simulink model "Comp_FDC_main"  (R2021b)
settings: Solver=FixedStepDiscrete  StartTime=0.0  StopTime=10.0  RelTol=1e-3  EnableMultiTasking=on
settings Model: DataDictionary=APPTypes.sldd  Creator=FVT23010  LastModifiedBy=FVT23010
settings SolverCC: AutoInsertRateTranBlk=on
settings DataIOCC: SaveFormat=StructureWithTime
settings OptimizationCC: DefaultParameterBehavior=Inlined  EnhancedBackFolding=on  PassReuseOutputArgsAs=Individual arguments  ZeroExternalMemoryAtStartup=off  ZeroInternalMemoryAtStartup=off  OptimizeBlockOrder=speed  DifferentSizesBufferReuse=on  OptimizationCustomize=off  EfficientTunableParamExpr=on
settings DebuggingCC: ParameterTunabilityLossMsg=error
settings ModelReferenceCC: ModelReferenceNumInstancesAllowed=Single
settings SFSimCC: MATLABDynamicMemAlloc=off
settings RTWCC: Description=AUTOSAR  SystemTargetFile=autosar.tlc  GenCodeOnly=on  TemplateMakefile=ert_default_tmf
settings CodeAppCC: ForceParamTrailComments=on  IgnoreCustomStorageClasses=off  OperatorAnnotations=on  SimulinkDataObjDesc=on  SFDataObjDesc=on  InsertBlockDesc=on
settings STFCustomTargetCC: TargetLangStandard=C99 (ISO)  MultiwordLength=256  ParMdlRefBuildCompliant=on  CompOptLevelCompliant=on  IncludeMdlTerminateFcn=off  CombineOutputUpdateFcns=on  SuppressErrorStatus=on  ERTCustomFileBanners=on  SupportNonFinite=off  SupportComplex=off  SupportContinuousTime=off  SupportNonInlinedSFcns=off  RemoveResetFunc=on  MATLABClassNameForMDSCustomization=Simulink.SoftwareTarget.ERTCustomization  AutosarCompliant=on  GRTInterface=off  UseToolchainInfoCompliant=on  LookupTableObjectStructAxisOrder=2,1,3,4,...  LUTObjectStructOrderEvenSpacing=Size,Table,Breakpoints  SystemTargetFile=autosar.tlc
settings ERTTargetCC: TargetLangStandard=C99 (ISO)  ConcurrentExecutionCompliant=off  IncludeMdlTerminateFcn=off  SuppressErrorStatus=on  SupportNonFinite=off  SupportComplex=off  ModelStepFunctionPrototypeControlCompliant=off  CPPClassGenCompliant=off  AutosarCompliant=on  LookupTableObjectStructAxisOrder=2,1,3,4,...  LUTObjectStructOrderEvenSpacing=Size,Table,Breakpoints  InlinedParameterPlacement=NonHierarchical  ERTCustomFileTemplate=example_file_process.tlc

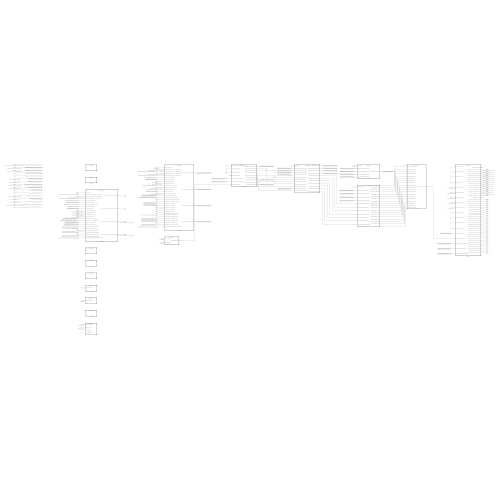
[thumbnail: Simulink's stored preview of the top-level diagram]
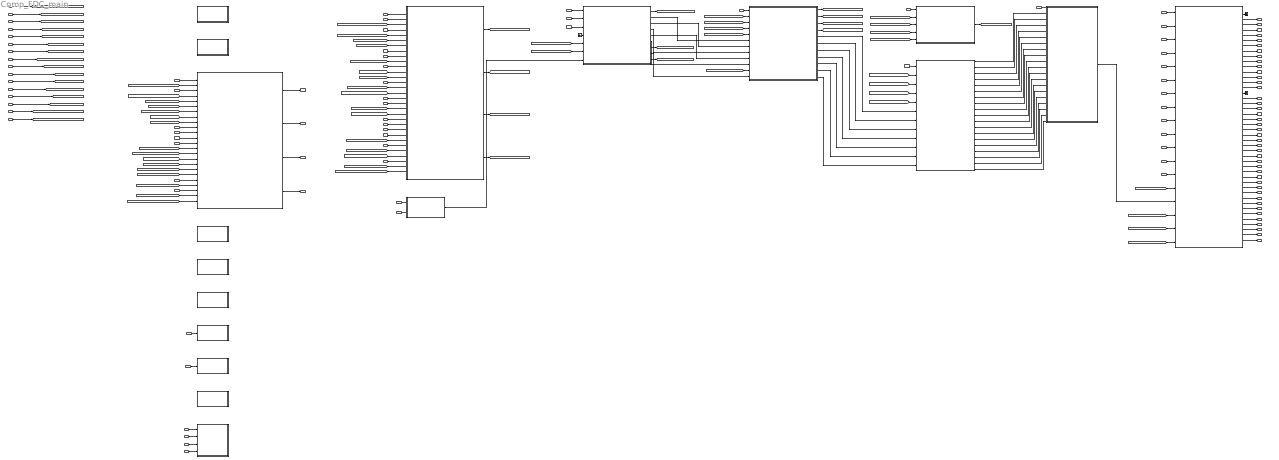
== system Comp_FDC_main ==
  run_SWC_CGW : Inport  OutputFunctionCall=on
  run_SWC_LOG_100ms : Inport  Port=2  SampleTime=0.1  OutputFunctionCall=on
  run_UARTConsole100ms : Inport  Port=3  SampleTime=0.1  OutputFunctionCall=on
  run_SWC_VES_1000ms : Inport  Port=4  SampleTime=1  OutputFunctionCall=on
  run_SWC_VES_IPCF_1ms : Inport  Port=5  SampleTime=0.001  OutputFunctionCall=on
  run_Trig_FwUpdate : Inport  Port=6  OutputFunctionCall=on
  run_Trig_IpcfDataReceive : Inport  Port=7  OutputFunctionCall=on
  run_SWC_HALIN_Rx_5ms : Inport  Port=8  SampleTime=0.005  OutputFunctionCall=on
  run_DKC_DataTask : Inport  Port=9  SampleTime=0.1  OutputFunctionCall=on
  run_DKC_MainTask : Inport  Port=10  SampleTime=0.01  OutputFunctionCall=on
  run_SWC_HALIN_CDD_IOEXPCDD_10ms : Inport  Port=11  SampleTime=0.01  OutputFunctionCall=on
  run_SWC_HALIN_CDD_Rx_10ms : Inport  Port=12  SampleTime=0.01  OutputFunctionCall=on
  run_SWC_HALIN_CDD_Rx_5ms : Inport  Port=13  SampleTime=0.005  OutputFunctionCall=on
  run_SWC_INP_5ms : Inport  Port=14  SampleTime=0.005  OutputFunctionCall=on
  run_SWC_SCP_5ms : Inport  Port=15  SampleTime=0.005  OutputFunctionCall=on
  run_SWC_FDC_RxTx_5ms : Inport  Port=16  SampleTime=0.005  OutputFunctionCall=on
  run_SWC_OUTP_5ms : Inport  Port=17  SampleTime=0.005  OutputFunctionCall=on
  run_SWC_HALOUT_PAS_1ms : Inport  Port=18  SampleTime=0.001  OutputFunctionCall=on
  run_SWC_HALOUT_UDS_10ms : Inport  Port=19  SampleTime=0.01  OutputFunctionCall=on
  run_SWC_HALOUT_Tx_5ms : Inport  Port=20  SampleTime=0.005  OutputFunctionCall=on
  run_SWC_HALOUT_Tx_10ms : Inport  Port=21  SampleTime=0.01  OutputFunctionCall=on
  run_SWC_HALOUT_Tx_80ms : Inport  Port=22  SampleTime=0.08  OutputFunctionCall=on
  run_SWC_HALOUT_Tx_5000ms : Inport  Port=23  SampleTime=5  OutputFunctionCall=on
  run_SWC_HALOUT_Tx_500ms : Inport  Port=24  SampleTime=0.5  OutputFunctionCall=on
  run_SWC_HALOUT_Tx_50ms : Inport  Port=25  SampleTime=0.05  OutputFunctionCall=on
  run_SWC_HALOUT_Tx_250ms : Inport  Port=26  SampleTime=0.25  OutputFunctionCall=on
  run_SWC_HALOUT_Tx_200ms : Inport  Port=27  SampleTime=0.2  OutputFunctionCall=on
  run_SWC_HALOUT_Tx_20ms : Inport  Port=28  SampleTime=0.02  OutputFunctionCall=on
  run_SWC_HALOUT_Tx_1000ms : Inport  Port=29  SampleTime=1  OutputFunctionCall=on
  run_SWC_HALOUT_Tx_100ms : Inport  Port=30  SampleTime=0.1  OutputFunctionCall=on
  HALR_CAN1_AC_BTMS_C1000_0_CAN1_SG_AC_BTMS_C1000_0 : Inport  Port=31  OutDataTypeStr=Bus: DT_CAN1_SG_AC_BTMS_C1000_0  PortDimensions=1  BusOutputAsStruct=on
  HALR_CAN1_AC_BTMS_C1000_1_CAN1_SG_AC_BTMS_C1000_1 : Inport  Port=32  OutDataTypeStr=Bus: DT_CAN1_SG_AC_BTMS_C1000_1  PortDimensions=1  BusOutputAsStruct=on
  HALR_CAN1_AC_BTMS_C1000_2_CAN1_SG_AC_BTMS_C1000_2 : Inport  Port=33  OutDataTypeStr=Bus: DT_CAN1_SG_AC_BTMS_C1000_2  PortDimensions=1  BusOutputAsStruct=on
  HALR_CAN1_AC_BTMS_C1000_4_CAN1_SG_AC_BTMS_C1000_4 : Inport  Port=34  OutDataTypeStr=Bus: DT_CAN1_SG_AC_BTMS_C1000_4  PortDimensions=1  BusOutputAsStruct=on
  HALR_CAN1_AC_BTMS_C5000_0_CAN1_SG_AC_BTMS_C5000_0 : Inport  Port=35  OutDataTypeStr=Bus: DT_CAN1_SG_AC_BTMS_C5000_0  PortDimensions=1  BusOutputAsStruct=on
  HALR_CAN1_ASC1_A_CAN1_SG_ASC1_A : Inport  Port=36  OutDataTypeStr=Bus: DT_CAN1_SG_ASC1_A  PortDimensions=1  BusOutputAsStruct=on
  HALR_CAN1_EBC1_CAN1_SG_EBC1 : Inport  Port=37  OutDataTypeStr=Bus: DT_CAN1_SG_EBC1  PortDimensions=1  BusOutputAsStruct=on
  HALR_CAN1_EBC2_CAN1_SG_EBC2 : Inport  Port=38  OutDataTypeStr=Bus: DT_CAN1_SG_EBC2  PortDimensions=1  BusOutputAsStruct=on
  HALR_CAN1_EBC5_CAN1_SG_EBC5 : Inport  Port=39  OutDataTypeStr=Bus: DT_CAN1_SG_EBC5  PortDimensions=1  BusOutputAsStruct=on
  HALR_CAN1_ECAS_DM1_CAN1_SG_ECAS_DM1 : Inport  Port=40  OutDataTypeStr=Bus: DT_CAN1_SG_ECAS_DM1  PortDimensions=1  BusOutputAsStruct=on
  HALR_CAN1_EMC1_EM1_CAN1_SG_EMC1_EM1 : Inport  Port=41  OutDataTypeStr=Bus: DT_CAN1_SG_EMC1_EM1  PortDimensions=1  BusOutputAsStruct=on
  HALR_CAN1_HRW_CAN1_SG_HRW : Inport  Port=42  OutDataTypeStr=Bus: DT_CAN1_SG_HRW  PortDimensions=1  BusOutputAsStruct=on
  HALR_CAN1_TC1_CAN1_SG_TC1 : Inport  Port=43  OutDataTypeStr=Bus: DT_CAN1_SG_TC1  PortDimensions=1  BusOutputAsStruct=on
  HALR_CAN1_TPMS1_CAN1_SG_TPMS1 : Inport  Port=44  OutDataTypeStr=Bus: DT_CAN1_SG_TPMS1  PortDimensions=1  BusOutputAsStruct=on
  HALR_CAN1_TPMS2_CAN1_SG_TPMS2 : Inport  Port=45  OutDataTypeStr=Bus: DT_CAN1_SG_TPMS2  PortDimensions=1  BusOutputAsStruct=on
  HALR_CAN1_TPMS3_CAN1_SG_TPMS3 : Inport  Port=46  OutDataTypeStr=Bus: DT_CAN1_SG_TPMS3  PortDimensions=1  BusOutputAsStruct=on
  HALR_CAN1_VDC1_CAN1_SG_VDC1 : Inport  Port=47  OutDataTypeStr=Bus: DT_CAN1_SG_VDC1  PortDimensions=1  BusOutputAsStruct=on
  HALR_CAN2_IVI_C100_0_CAN2_SG_IVI_C100_0 : Inport  Port=48  OutDataTypeStr=Bus: DT_CAN2_SG_IVI_C100_0  PortDimensions=1  BusOutputAsStruct=on
  HALR_CAN3_B2TM_Info_CAN3_SG_B2TM_Info : Inport  Port=49  OutDataTypeStr=Bus: DT_CAN3_SG_B2TM_Info  PortDimensions=1  BusOutputAsStruct=on
  HALR_CAN3_B2V_BattInfo1_CAN3_SG_B2V_BattInfo1 : Inport  Port=50  OutDataTypeStr=Bus: DT_CAN3_SG_B2V_BattInfo1  PortDimensions=1  BusOutputAsStruct=on
  HALR_CAN3_B2V_CurrentLimit_CAN3_SG_B2V_CurrentLimit : Inport  Port=51  OutDataTypeStr=Bus: DT_CAN3_SG_B2V_CurrentLimit  PortDimensions=1  BusOutputAsStruct=on
  HALR_CAN3_B2V_Fult1_32960_CAN3_SG_B2V_Fult1_32960 : Inport  Port=52  OutDataTypeStr=Bus: DT_CAN3_SG_B2V_Fult1_32960  PortDimensions=1  BusOutputAsStruct=on
  HALR_CAN3_B2V_ST1_CAN3_SG_B2V_ST1 : Inport  Port=53  OutDataTypeStr=Bus: DT_CAN3_SG_B2V_ST1  PortDimensions=1  BusOutputAsStruct=on
  HALR_CAN3_B2V_ST2_CAN3_SG_B2V_ST2 : Inport  Port=54  OutDataTypeStr=Bus: DT_CAN3_SG_B2V_ST2  PortDimensions=1  BusOutputAsStruct=on
  HALR_CAN3_B2V_ST4_CAN3_SG_B2V_ST4 : Inport  Port=55  OutDataTypeStr=Bus: DT_CAN3_SG_B2V_ST4  PortDimensions=1  BusOutputAsStruct=on
  HALR_CAN3_B2V_ST5_CAN3_SG_B2V_ST5 : Inport  Port=56  OutDataTypeStr=Bus: DT_CAN3_SG_B2V_ST5  PortDimensions=1  BusOutputAsStruct=on
  HALR_CAN3_EWP1_CAN3_SG_EWP1 : Inport  Port=57  OutDataTypeStr=Bus: DT_CAN3_SG_EWP1  PortDimensions=1  BusOutputAsStruct=on
  HALR_CAN3_TM_MCUSta1_CAN3_SG_TM_MCUSta1 : Inport  Port=58  OutDataTypeStr=Bus: DT_CAN3_SG_TM_MCUSta1  PortDimensions=1  BusOutputAsStruct=on
  HALR_CAN3_TM_MCUSta2_CAN3_SG_TM_MCUSta2 : Inport  Port=59  OutDataTypeStr=Bus: DT_CAN3_SG_TM_MCUSta2  PortDimensions=1  BusOutputAsStruct=on
  HALR_CAN3_TM_MCUSta3_CAN3_SG_TM_MCUSta3 : Inport  Port=60  OutDataTypeStr=Bus: DT_CAN3_SG_TM_MCUSta3  PortDimensions=1  BusOutputAsStruct=on
  HALR_CAN4_ZFR_C100_0_CAN4_SG_ZFR_C100_0 : Inport  Port=61  OutDataTypeStr=Bus: DT_CAN4_SG_ZFR_C100_0  PortDimensions=1  BusOutputAsStruct=on
  HALR_CAN4_ZFR_C5000_0_CAN4_SG_ZFR_C5000_0 : Inport  Port=62  OutDataTypeStr=Bus: DT_CAN4_SG_ZFR_C5000_0  PortDimensions=1  BusOutputAsStruct=on
  HALR_CAN4_ZFR_CE100_0_CAN4_SG_ZFR_CE100_0 : Inport  Port=63  OutDataTypeStr=Bus: DT_CAN4_SG_ZFR_CE100_0  PortDimensions=1  BusOutputAsStruct=on
  HALR_CAN4_ZRR_C5000_0_CAN4_SG_ZRR_C5000_0 : Inport  Port=64  OutDataTypeStr=Bus: DT_CAN4_SG_ZRR_C5000_0  PortDimensions=1  BusOutputAsStruct=on
  HALR_CAN4_ZRR_CE100_0_CAN4_SG_ZRR_CE100_0 : Inport  Port=65  OutDataTypeStr=Bus: DT_CAN4_SG_ZRR_CE100_0  PortDimensions=1  BusOutputAsStruct=on
  HALR_CAN4_ZRR_CE100_1_CAN4_SG_ZRR_CE100_1 : Inport  Port=66  OutDataTypeStr=Bus: DT_CAN4_SG_ZRR_CE100_1  PortDimensions=1  BusOutputAsStruct=on
  HALR_CAN4_zGW_CANRr1_C50_0_CAN4_SG_zGW_CANRr1_C50_0 : Inport  Port=67  OutDataTypeStr=Bus: DT_CAN4_SG_zGW_CANRr1_C50_0  PortDimensions=1  BusOutputAsStruct=on
  Ground_1 : Ground
  SWC_APS : ModelReference  ModelNameDialog=SWC_APS_type  SimulationMode=Normal  ScheduleRates=on  ModelReferenceVersion=1.1
  SWC_CDD : ModelReference  ModelNameDialog=SWC_CDD_type  SimulationMode=Normal  ScheduleRates=on  ModelReferenceVersion=1.1
  SWC_CGW : ModelReference  ModelNameDialog=SWC_CGW_type  SimulationMode=Normal  ScheduleRates=on  ModelReferenceVersion=1.1
  SWC_DID : ModelReference  ModelNameDialog=SWC_DID_type  SimulationMode=Normal  ScheduleRates=on  ModelReferenceVersion=1.1
  SWC_DKC : ModelReference  ModelNameDialog=SWC_DKC_type  SimulationMode=Normal  ScheduleRates=on  ModelReferenceVersion=1.1
  SWC_FDC : ModelReference  ModelNameDialog=SWC_FDC_type  SimulationMode=Normal  ScheduleRates=on  ModelReferenceVersion=1.1
  SWC_HALIN : ModelReference  ModelNameDialog=SWC_HALIN_type  SimulationMode=Normal  ScheduleRates=on  ModelReferenceVersion=1.1
  SWC_HALIN_CDD : ModelReference  ModelNameDialog=SWC_HALIN_CDD_type  SimulationMode=Normal  ScheduleRates=on  ModelReferenceVersion=1.1
  SWC_HALOUT : ModelReference  ModelNameDialog=SWC_HALOUT_type  SimulationMode=Normal  ScheduleRates=on  ModelReferenceVersion=1.1
  SWC_IMU : ModelReference  ModelNameDialog=SWC_IMU_type  SimulationMode=Normal  ScheduleRates=on  ModelReferenceVersion=1.1
  SWC_INP : ModelReference  ModelNameDialog=SWC_INP_type  SimulationMode=Normal  ScheduleRates=on  ModelReferenceVersion=1.1
  SWC_IOEXP : ModelReference  ModelNameDialog=SWC_IOEXP_type  SimulationMode=Normal  ScheduleRates=on  ModelReferenceVersion=1.1
  SWC_LOG : ModelReference  ModelNameDialog=SWC_LOG_type  SimulationMode=Normal  ScheduleRates=on  ModelReferenceVersion=1.1
  SWC_OUTP : ModelReference  ModelNameDialog=SWC_OUTP_type  SimulationMode=Normal  ScheduleRates=on  ModelReferenceVersion=1.1
  SWC_SCP : ModelReference  ModelNameDialog=SWC_SCP_type  SimulationMode=Normal  ScheduleRates=on  ModelReferenceVersion=1.1
  SWC_UART : ModelReference  ModelNameDialog=SWC_UART_type  SimulationMode=Normal  ScheduleRates=on  ModelReferenceVersion=1.1
  SWC_UDS : ModelReference  ModelNameDialog=SWC_UDS_type  SimulationMode=Normal  ScheduleRates=on  ModelReferenceVersion=1.1
  SWC_VES : ModelReference  ModelNameDialog=SWC_VES_type  SimulationMode=Normal  ScheduleRates=on  ModelReferenceVersion=1.1
  Terminator_1 : Terminator
  Terminator_2 : Terminator
  HALP_CAN1_CGW_FD1_C100_3_CAN1_SG_CGW_FD1_C100_3 : Outport  OutDataTypeStr=Bus: DT_CAN1_SG_CGW_FD1_C100_3  PortDimensions=1  BusOutputAsStruct=on
  HALP_CAN1_FD1_C1000_0_CAN1_SG_FD1_C1000_0 : Outport  Port=2  OutDataTypeStr=Bus: DT_CAN1_SG_FD1_C1000_0  PortDimensions=1  BusOutputAsStruct=on
  HALP_CAN1_FD1_C100_0_CAN1_SG_FD1_C100_0 : Outport  Port=3  OutDataTypeStr=Bus: DT_CAN1_SG_FD1_C100_0  PortDimensions=1  BusOutputAsStruct=on
  HALP_CAN1_FD1_C100_1_CAN1_SG_FD1_C100_1 : Outport  Port=4  OutDataTypeStr=Bus: DT_CAN1_SG_FD1_C100_1  PortDimensions=1  BusOutputAsStruct=on
  HALP_CAN1_FD1_C100_2_CAN1_SG_FD1_C100_2 : Outport  Port=5  OutDataTypeStr=Bus: DT_CAN1_SG_FD1_C100_2  PortDimensions=1  BusOutputAsStruct=on
  HALP_CAN1_FD1_C100_3_CAN1_SG_FD1_C100_3 : Outport  Port=6  OutDataTypeStr=Bus: DT_CAN1_SG_FD1_C100_3  PortDimensions=1  BusOutputAsStruct=on
  HALP_CAN1_FD1_C10_0_CAN1_SG_FD1_C10_0 : Outport  Port=7  OutDataTypeStr=Bus: DT_CAN1_SG_FD1_C10_0  PortDimensions=1  BusOutputAsStruct=on
  HALP_CAN1_FD1_C10_1_CAN1_SG_FD1_C10_1 : Outport  Port=8  OutDataTypeStr=Bus: DT_CAN1_SG_FD1_C10_1  PortDimensions=1  BusOutputAsStruct=on
  HALP_CAN1_FD1_C200_0_CAN1_SG_FD1_C200_0 : Outport  Port=9  OutDataTypeStr=Bus: DT_CAN1_SG_FD1_C200_0  PortDimensions=1  BusOutputAsStruct=on
  HALP_CAN1_FD1_C20_0_CAN1_SG_FD1_C20_0 : Outport  Port=10  OutDataTypeStr=Bus: DT_CAN1_SG_FD1_C20_0  PortDimensions=1  BusOutputAsStruct=on
  HALP_CAN1_FD1_C250_0_CAN1_SG_FD1_C250_0 : Outport  Port=11  OutDataTypeStr=Bus: DT_CAN1_SG_FD1_C250_0  PortDimensions=1  BusOutputAsStruct=on
  HALP_CAN1_FD1_C5000_0_CAN1_SG_FD1_C5000_0 : Outport  Port=12  OutDataTypeStr=Bus: DT_CAN1_SG_FD1_C5000_0  PortDimensions=1  BusOutputAsStruct=on
  HALP_CAN1_FD1_C5000_1_CAN1_SG_FD1_C5000_1 : Outport  Port=13  OutDataTypeStr=Bus: DT_CAN1_SG_FD1_C5000_1  PortDimensions=1  BusOutputAsStruct=on
  HALP_CAN1_FD1_C50_0_CAN1_SG_FD1_C50_0 : Outport  Port=14  OutDataTypeStr=Bus: DT_CAN1_SG_FD1_C50_0  PortDimensions=1  BusOutputAsStruct=on
  HALP_CAN1_FD1_C50_1_CAN1_SG_FD1_C50_1 : Outport  Port=15  OutDataTypeStr=Bus: DT_CAN1_SG_FD1_C50_1  PortDimensions=1  BusOutputAsStruct=on
  HALP_CAN1_FD1_C80_0_CAN1_SG_FD1_C80_0 : Outport  Port=16  OutDataTypeStr=Bus: DT_CAN1_SG_FD1_C80_0  PortDimensions=1  BusOutputAsStruct=on
  HALP_CAN1_FD1_CE100_0_CAN1_SG_FD1_CE100_0 : Outport  Port=17  OutDataTypeStr=Bus: DT_CAN1_SG_FD1_CE100_0  PortDimensions=1  BusOutputAsStruct=on
  HALP_CAN1_FD1_CE100_1_CAN1_SG_FD1_CE100_1 : Outport  Port=18  OutDataTypeStr=Bus: DT_CAN1_SG_FD1_CE100_1  PortDimensions=1  BusOutputAsStruct=on
  HALP_CAN1_FD1_CE100_2_CAN1_SG_FD1_CE100_2 : Outport  Port=19  OutDataTypeStr=Bus: DT_CAN1_SG_FD1_CE100_2  PortDimensions=1  BusOutputAsStruct=on
  HALP_CAN2_CGW_FD2_C1000_0_CAN2_SG_CGW_FD2_C1000_0 : Outport  Port=20  OutDataTypeStr=Bus: DT_CAN2_SG_CGW_FD2_C1000_0  PortDimensions=1  BusOutputAsStruct=on
  HALP_CAN2_CGW_GW2_C100_0_CAN2_SG_CGW_GW2_C100_0 : Outport  Port=21  OutDataTypeStr=Bus: DT_CAN2_SG_CGW_GW2_C100_0  PortDimensions=1  BusOutputAsStruct=on
  HALP_CAN2_FD2_C1000_0_CAN2_SG_FD2_C1000_0 : Outport  Port=22  OutDataTypeStr=Bus: DT_CAN2_SG_FD2_C1000_0  PortDimensions=1  BusOutputAsStruct=on
  HALP_CAN2_FD2_C10_0_CAN2_SG_FD2_C10_0 : Outport  Port=23  OutDataTypeStr=Bus: DT_CAN2_SG_FD2_C10_0  PortDimensions=1  BusOutputAsStruct=on
  HALP_CAN2_FD2_C200_0_CAN2_SG_FD2_C200_0 : Outport  Port=24  OutDataTypeStr=Bus: DT_CAN2_SG_FD2_C200_0  PortDimensions=1  BusOutputAsStruct=on
  HALP_CAN2_FD2_C500_0_CAN2_SG_FD2_C500_0 : Outport  Port=25  OutDataTypeStr=Bus: DT_CAN2_SG_FD2_C500_0  PortDimensions=1  BusOutputAsStruct=on
  HALP_CAN2_FD2_C50_0_CAN2_SG_FD2_C50_0 : Outport  Port=26  OutDataTypeStr=Bus: DT_CAN2_SG_FD2_C50_0  PortDimensions=1  BusOutputAsStruct=on
  HALP_CAN2_FD2_CE100_0_CAN2_SG_FD2_CE100_0 : Outport  Port=27  OutDataTypeStr=Bus: DT_CAN2_SG_FD2_CE100_0  PortDimensions=1  BusOutputAsStruct=on
  HALP_CAN2_GW2_C100_0_CAN2_SG_GW2_C100_0 : Outport  Port=28  OutDataTypeStr=Bus: DT_CAN2_SG_GW2_C100_0  PortDimensions=1  BusOutputAsStruct=on
  HALP_CAN3_FD3_C100_0_CAN3_SG_FD3_C100_0 : Outport  Port=29  OutDataTypeStr=Bus: DT_CAN3_SG_FD3_C100_0  PortDimensions=1  BusOutputAsStruct=on
  HALP_CAN3_FD3_C10_0_CAN3_SG_FD3_C10_0 : Outport  Port=30  OutDataTypeStr=Bus: DT_CAN3_SG_FD3_C10_0  PortDimensions=1  BusOutputAsStruct=on
  HALP_CAN3_FD3_C10_1_CAN3_SG_FD3_C10_1 : Outport  Port=31  OutDataTypeStr=Bus: DT_CAN3_SG_FD3_C10_1  PortDimensions=1  BusOutputAsStruct=on
  HALP_CAN3_FD3_C200_0_CAN3_SG_FD3_C200_0 : Outport  Port=32  OutDataTypeStr=Bus: DT_CAN3_SG_FD3_C200_0  PortDimensions=1  BusOutputAsStruct=on
  HALP_CAN3_FD3_C200_1_CAN3_SG_FD3_C200_1 : Outport  Port=33  OutDataTypeStr=Bus: DT_CAN3_SG_FD3_C200_1  PortDimensions=1  BusOutputAsStruct=on
  HALP_CAN4_FD4_C100_0_CAN4_SG_FD4_C100_0 : Outport  Port=34  OutDataTypeStr=Bus: DT_CAN4_SG_FD4_C100_0  PortDimensions=1  BusOutputAsStruct=on
  HALP_CAN4_FD4_C10_0_CAN4_SG_FD4_C10_0 : Outport  Port=35  OutDataTypeStr=Bus: DT_CAN4_SG_FD4_C10_0  PortDimensions=1  BusOutputAsStruct=on
  HALP_CAN4_FD4_C200_0_CAN4_SG_FD4_C200_0 : Outport  Port=36  OutDataTypeStr=Bus: DT_CAN4_SG_FD4_C200_0  PortDimensions=1  BusOutputAsStruct=on
  HALP_CAN4_FD4_CE100_0_CAN4_SG_FD4_CE100_0 : Outport  Port=37  OutDataTypeStr=Bus: DT_CAN4_SG_FD4_CE100_0  PortDimensions=1  BusOutputAsStruct=on
  HALP_CAN4_FD4_CE100_1_CAN4_SG_FD4_CE100_1 : Outport  Port=38  OutDataTypeStr=Bus: DT_CAN4_SG_FD4_CE100_1  PortDimensions=1  BusOutputAsStruct=on
  HALP_CAN5_FD5_C100_0_CAN5_SG_FD5_C100_0 : Outport  Port=39  OutDataTypeStr=Bus: DT_CAN5_SG_FD5_C100_0  PortDimensions=1  BusOutputAsStruct=on
  HALP_CAN5_FD5_C200_0_CAN5_SG_FD5_C200_0 : Outport  Port=40  OutDataTypeStr=Bus: DT_CAN5_SG_FD5_C200_0  PortDimensions=1  BusOutputAsStruct=on
  HALP_CAN6_FD6_C200_0_CAN6_SG_FD6_C200_0 : Outport  Port=41  OutDataTypeStr=Bus: DT_CAN6_SG_FD6_C200_0  PortDimensions=1  BusOutputAsStruct=on
  HALP_CAN7_FD7_C100_0_CAN7_SG_FD7_C100_0 : Outport  Port=42  OutDataTypeStr=Bus: DT_CAN7_SG_FD7_C100_0  PortDimensions=1  BusOutputAsStruct=on
  HALP_CAN7_FD7_C10_0_CAN7_SG_FD7_C10_0 : Outport  Port=43  OutDataTypeStr=Bus: DT_CAN7_SG_FD7_C10_0  PortDimensions=1  BusOutputAsStruct=on
  HALP_CAN7_FD7_C200_0_CAN7_SG_FD7_C200_0 : Outport  Port=44  OutDataTypeStr=Bus: DT_CAN7_SG_FD7_C200_0  PortDimensions=1  BusOutputAsStruct=on
  HALP_CAN7_FD7_C50_0_CAN7_SG_FD7_C50_0 : Outport  Port=45  OutDataTypeStr=Bus: DT_CAN7_SG_FD7_C50_0  PortDimensions=1  BusOutputAsStruct=on
  HALP_CAN7_FD7_CE100_0_CAN7_SG_FD7_CE100_0 : Outport  Port=46  OutDataTypeStr=Bus: DT_CAN7_SG_FD7_CE100_0  PortDimensions=1  BusOutputAsStruct=on
  wires:
  run_SWC_CGW/1 -> SWC_CGW/1
  run_SWC_LOG_100ms/1 -> SWC_LOG/1
  run_UARTConsole100ms/1 -> SWC_UART/1
  run_SWC_VES_1000ms/1 -> SWC_VES/1
  run_SWC_VES_IPCF_1ms/1 -> SWC_VES/2
  run_Trig_FwUpdate/1 -> SWC_VES/3
  run_Trig_IpcfDataReceive/1 -> SWC_VES/4
  run_SWC_HALIN_Rx_5ms/1 -> SWC_HALIN/1
  run_DKC_DataTask/1 -> SWC_DKC/1
  run_DKC_MainTask/1 -> SWC_DKC/2
  run_SWC_HALIN_CDD_IOEXPCDD_10ms/1 -> SWC_HALIN_CDD/1
  run_SWC_HALIN_CDD_Rx_10ms/1 -> SWC_HALIN_CDD/2
  run_SWC_HALIN_CDD_Rx_5ms/1 -> SWC_HALIN_CDD/3
  run_SWC_INP_5ms/1 -> SWC_INP/1
  run_SWC_SCP_5ms/1 -> SWC_SCP/1
  run_SWC_FDC_RxTx_5ms/1 -> SWC_FDC/1
  run_SWC_OUTP_5ms/1 -> SWC_OUTP/1
  run_SWC_HALOUT_PAS_1ms/1 -> SWC_HALOUT/1
  run_SWC_HALOUT_UDS_10ms/1 -> SWC_HALOUT/2
  run_SWC_HALOUT_Tx_5ms/1 -> SWC_HALOUT/3
  run_SWC_HALOUT_Tx_10ms/1 -> SWC_HALOUT/4
  run_SWC_HALOUT_Tx_80ms/1 -> SWC_HALOUT/5
  run_SWC_HALOUT_Tx_5000ms/1 -> SWC_HALOUT/6
  run_SWC_HALOUT_Tx_500ms/1 -> SWC_HALOUT/7
  run_SWC_HALOUT_Tx_50ms/1 -> SWC_HALOUT/8
  run_SWC_HALOUT_Tx_250ms/1 -> SWC_HALOUT/9
  run_SWC_HALOUT_Tx_200ms/1 -> SWC_HALOUT/10
  run_SWC_HALOUT_Tx_20ms/1 -> SWC_HALOUT/11
  run_SWC_HALOUT_Tx_1000ms/1 -> SWC_HALOUT/12
  run_SWC_HALOUT_Tx_100ms/1 -> SWC_HALOUT/13
  HALR_CAN1_AC_BTMS_C1000_0_CAN1_SG_AC_BTMS_C1000_0/1 -> SWC_HALIN/2
  HALR_CAN1_AC_BTMS_C1000_4_CAN1_SG_AC_BTMS_C1000_4/1 -> SWC_HALIN/4
  HALR_CAN1_EBC2_CAN1_SG_EBC2/1 -> SWC_HALIN/8
  HALR_CAN1_EBC5_CAN1_SG_EBC5/1 -> SWC_HALIN/9
  HALR_CAN1_EMC1_EM1_CAN1_SG_EMC1_EM1/1 -> SWC_HALIN/11
  HALR_CAN2_IVI_C100_0_CAN2_SG_IVI_C100_0/1 -> SWC_HALIN/14
  HALR_CAN3_B2V_CurrentLimit_CAN3_SG_B2V_CurrentLimit/1 -> SWC_HALIN/17
  HALR_CAN3_B2V_Fult1_32960_CAN3_SG_B2V_Fult1_32960/1 -> SWC_HALIN/18
  HALR_CAN3_B2V_ST4_CAN3_SG_B2V_ST4/1 -> SWC_HALIN/21
  HALR_CAN3_B2V_ST5_CAN3_SG_B2V_ST5/1 -> SWC_HALIN/22
  HALR_CAN3_EWP1_CAN3_SG_EWP1/1 -> SWC_HALIN/23
  HALR_CAN3_TM_MCUSta1_CAN3_SG_TM_MCUSta1/1 -> SWC_HALIN/24
  HALR_CAN3_TM_MCUSta3_CAN3_SG_TM_MCUSta3/1 -> SWC_HALIN/26
  HALR_CAN4_ZRR_CE100_0_CAN4_SG_ZRR_CE100_0/1 -> SWC_HALIN/29
  HALR_CAN1_AC_BTMS_C1000_2_CAN1_SG_AC_BTMS_C1000_2/1 -> SWC_CGW/3
  HALR_CAN1_TPMS1_CAN1_SG_TPMS1/1 -> SWC_CGW/10
  HALR_CAN1_TPMS2_CAN1_SG_TPMS2/1 -> SWC_CGW/11
  HALR_CAN1_TPMS3_CAN1_SG_TPMS3/1 -> SWC_CGW/12
  HALR_CAN1_VDC1_CAN1_SG_VDC1/1 -> SWC_CGW/13
  HALR_CAN4_ZFR_C5000_0_CAN4_SG_ZFR_C5000_0/1 -> SWC_CGW/20
  HALR_CAN4_ZRR_C5000_0_CAN4_SG_ZRR_C5000_0/1 -> SWC_CGW/22
  SWC_HALOUT/36 -> HALP_CAN1_FD1_C100_0_CAN1_SG_FD1_C100_0/1
  SWC_HALOUT/37 -> HALP_CAN1_FD1_C100_1_CAN1_SG_FD1_C100_1/1
  SWC_HALOUT/38 -> HALP_CAN1_FD1_C100_2_CAN1_SG_FD1_C100_2/1
  SWC_HALOUT/39 -> HALP_CAN1_FD1_C100_3_CAN1_SG_FD1_C100_3/1
  SWC_HALOUT/9 -> HALP_CAN1_FD1_C10_0_CAN1_SG_FD1_C10_0/1
  SWC_HALOUT/10 -> HALP_CAN1_FD1_C10_1_CAN1_SG_FD1_C10_1/1
  SWC_HALOUT/26 -> HALP_CAN1_FD1_C200_0_CAN1_SG_FD1_C200_0/1
  SWC_HALOUT/34 -> HALP_CAN1_FD1_C20_0_CAN1_SG_FD1_C20_0/1
  SWC_HALOUT/25 -> HALP_CAN1_FD1_C250_0_CAN1_SG_FD1_C250_0/1
  SWC_HALOUT/18 -> HALP_CAN1_FD1_C5000_0_CAN1_SG_FD1_C5000_0/1
  SWC_HALOUT/19 -> HALP_CAN1_FD1_C5000_1_CAN1_SG_FD1_C5000_1/1
  SWC_HALOUT/21 -> HALP_CAN1_FD1_C50_0_CAN1_SG_FD1_C50_0/1
  SWC_HALOUT/22 -> HALP_CAN1_FD1_C50_1_CAN1_SG_FD1_C50_1/1
  SWC_HALOUT/17 -> HALP_CAN1_FD1_C80_0_CAN1_SG_FD1_C80_0/1
  SWC_HALOUT/7 -> HALP_CAN1_FD1_CE100_0_CAN1_SG_FD1_CE100_0/1
  SWC_HALOUT/8 -> HALP_CAN1_FD1_CE100_1_CAN1_SG_FD1_CE100_1/1
  SWC_HALOUT/2 -> HALP_CAN1_FD1_CE100_2_CAN1_SG_FD1_CE100_2/1
  SWC_HALOUT/35 -> HALP_CAN2_FD2_C1000_0_CAN2_SG_FD2_C1000_0/1
  SWC_HALOUT/11 -> HALP_CAN2_FD2_C10_0_CAN2_SG_FD2_C10_0/1
  SWC_HALOUT/27 -> HALP_CAN2_FD2_C200_0_CAN2_SG_FD2_C200_0/1
  SWC_HALOUT/20 -> HALP_CAN2_FD2_C500_0_CAN2_SG_FD2_C500_0/1
  SWC_HALOUT/23 -> HALP_CAN2_FD2_C50_0_CAN2_SG_FD2_C50_0/1
  SWC_HALOUT/3 -> HALP_CAN2_FD2_CE100_0_CAN2_SG_FD2_CE100_0/1
  SWC_HALOUT/40 -> HALP_CAN2_GW2_C100_0_CAN2_SG_GW2_C100_0/1
  SWC_HALOUT/41 -> HALP_CAN3_FD3_C100_0_CAN3_SG_FD3_C100_0/1
  SWC_HALOUT/12 -> HALP_CAN3_FD3_C10_0_CAN3_SG_FD3_C10_0/1
  SWC_HALOUT/13 -> HALP_CAN3_FD3_C10_1_CAN3_SG_FD3_C10_1/1
  SWC_HALOUT/28 -> HALP_CAN3_FD3_C200_0_CAN3_SG_FD3_C200_0/1
  SWC_HALOUT/29 -> HALP_CAN3_FD3_C200_1_CAN3_SG_FD3_C200_1/1
  SWC_HALOUT/42 -> HALP_CAN4_FD4_C100_0_CAN4_SG_FD4_C100_0/1
  SWC_HALOUT/14 -> HALP_CAN4_FD4_C10_0_CAN4_SG_FD4_C10_0/1
  SWC_HALOUT/30 -> HALP_CAN4_FD4_C200_0_CAN4_SG_FD4_C200_0/1
  SWC_HALOUT/4 -> HALP_CAN4_FD4_CE100_0_CAN4_SG_FD4_CE100_0/1
  SWC_HALOUT/5 -> HALP_CAN4_FD4_CE100_1_CAN4_SG_FD4_CE100_1/1
  SWC_HALOUT/43 -> HALP_CAN5_FD5_C100_0_CAN5_SG_FD5_C100_0/1
  SWC_HALOUT/31 -> HALP_CAN5_FD5_C200_0_CAN5_SG_FD5_C200_0/1
  SWC_HALOUT/32 -> HALP_CAN6_FD6_C200_0_CAN6_SG_FD6_C200_0/1
  SWC_HALOUT/44 -> HALP_CAN7_FD7_C100_0_CAN7_SG_FD7_C100_0/1
  SWC_HALOUT/15 -> HALP_CAN7_FD7_C10_0_CAN7_SG_FD7_C10_0/1
  SWC_HALOUT/33 -> HALP_CAN7_FD7_C200_0_CAN7_SG_FD7_C200_0/1
  SWC_HALOUT/24 -> HALP_CAN7_FD7_C50_0_CAN7_SG_FD7_C50_0/1
  SWC_HALOUT/6 -> HALP_CAN7_FD7_CE100_0_CAN7_SG_FD7_CE100_0/1
  SWC_CGW/1 -> HALP_CAN1_FD1_C1000_0_CAN1_SG_FD1_C1000_0/1
  SWC_CGW/2 -> HALP_CAN1_CGW_FD1_C100_3_CAN1_SG_CGW_FD1_C100_3/1
  SWC_CGW/3 -> HALP_CAN2_CGW_FD2_C1000_0_CAN2_SG_CGW_FD2_C1000_0/1
  SWC_CGW/4 -> HALP_CAN2_CGW_GW2_C100_0_CAN2_SG_CGW_GW2_C100_0/1
  SWC_DKC/1 -> SWC_HALIN_CDD/7
  SWC_HALIN_CDD/2 -> SWC_INP/6
  SWC_HALIN_CDD/3 -> SWC_INP/7
  SWC_HALIN_CDD/4 -> SWC_INP/8
  SWC_HALIN_CDD/5 -> SWC_INP/9
  SWC_HALIN_CDD/6 -> SWC_INP/10
  SWC_HALIN_CDD/8 -> SWC_INP/12
  SWC_INP/5 -> SWC_FDC/6
  SWC_INP/6 -> SWC_FDC/7
  SWC_INP/7 -> SWC_FDC/8
  SWC_INP/8 -> SWC_FDC/9
  SWC_INP/9 -> SWC_FDC/10
  SWC_INP/10 -> SWC_FDC/11
  SWC_INP/11 -> SWC_FDC/12
  SWC_FDC/1 -> SWC_OUTP/2
  SWC_FDC/2 -> SWC_OUTP/3
  SWC_FDC/3 -> SWC_OUTP/4
  SWC_FDC/4 -> SWC_OUTP/5
  SWC_FDC/5 -> SWC_OUTP/6
  SWC_FDC/7 -> SWC_OUTP/8
  SWC_FDC/8 -> SWC_OUTP/9
  SWC_FDC/9 -> SWC_OUTP/10
  SWC_FDC/10 -> SWC_OUTP/11
  SWC_FDC/11 -> SWC_OUTP/12
  SWC_FDC/12 -> SWC_OUTP/13
  SWC_FDC/13 -> SWC_OUTP/14
  SWC_FDC/14 -> SWC_OUTP/15
  SWC_FDC/15 -> SWC_OUTP/16
  SWC_FDC/16 -> SWC_OUTP/17
  SWC_FDC/17 -> SWC_OUTP/18
  SWC_FDC/18 -> SWC_OUTP/19
  SWC_FDC/19 -> SWC_OUTP/20
  SWC_FDC/6 -> SWC_OUTP/7
  SWC_OUTP/1 -> SWC_HALOUT/15
  SWC_SCP/1 -> [P_BSCP_outputs_BSCP_outputs_Tag]
  [P_BSCP_outputs_BSCP_outputs_Tag] -> SWC_HALOUT/14
  SWC_HALIN_CDD/1 -> [P_NVMReadCDD_u8Array1024_NVMReadData_Tag]
  [P_NVMReadCDD_u8Array1024_NVMReadData_Tag] -> SWC_HALOUT/18
  SWC_HALIN_CDD/9 -> [P_BHAL_DID_outputs_BHAL_DID_outputs_Tag]
  [P_BHAL_DID_outputs_BHAL_DID_outputs_Tag] -> SWC_HALOUT/17
  SWC_INP/4 -> [P_BINP_CAN4_outputs_BINP_CAN4_outputs_Tag]
  [P_BINP_CAN4_outputs_BINP_CAN4_outputs_Tag] -> SWC_FDC/5
  [P_BINP_CAN4_outputs_BINP_CAN4_outputs_Tag] -> SWC_SCP/5
  SWC_INP/3 -> [P_BINP_CAN3_outputs_BINP_CAN3_outputs_Tag]
  [P_BINP_CAN3_outputs_BINP_CAN3_outputs_Tag] -> SWC_FDC/4
  [P_BINP_CAN3_outputs_BINP_CAN3_outputs_Tag] -> SWC_SCP/4
  SWC_INP/2 -> [P_BINP_CAN2_outputs_BINP_CAN2_outputs_Tag]
  [P_BINP_CAN2_outputs_BINP_CAN2_outputs_Tag] -> SWC_FDC/3
  [P_BINP_CAN2_outputs_BINP_CAN2_outputs_Tag] -> SWC_SCP/3
  SWC_INP/1 -> [P_BINP_CAN1_outputs_BINP_CAN1_outputs_Tag]
  [P_BINP_CAN1_outputs_BINP_CAN1_outputs_Tag] -> SWC_FDC/2
  [P_BINP_CAN1_outputs_BINP_CAN1_outputs_Tag] -> SWC_SCP/2
  SWC_HALIN_CDD/7 -> [P_BHAL_SYS_outputs_BHAL_SYS_outputs_Tag]
  [P_BHAL_SYS_outputs_BHAL_SYS_outputs_Tag] -> SWC_INP/11
  [P_BHAL_SYS_outputs_BHAL_SYS_outputs_Tag] -> SWC_HALOUT/16
  SWC_HALIN/3 -> [P_BHAL_CAN3_outputs_BHAL_CAN3_outputs_Tag]
  [P_BHAL_CAN3_outputs_BHAL_CAN3_outputs_Tag] -> SWC_INP/4
  SWC_HALIN/1 -> [P_BHAL_CAN1_outputs_BHAL_CAN1_outputs_Tag]
  [P_BHAL_CAN1_outputs_BHAL_CAN1_outputs_Tag] -> SWC_INP/2
  SWC_HALIN/4 -> [P_BHAL_CAN4_outputs_BHAL_CAN4_outputs_Tag]
  [P_BHAL_CAN4_outputs_BHAL_CAN4_outputs_Tag] -> SWC_HALIN_CDD/6
  [P_BHAL_CAN4_outputs_BHAL_CAN4_outputs_Tag] -> SWC_INP/5
  SWC_HALIN/2 -> [P_BHAL_CAN2_outputs_BHAL_CAN2_outputs_Tag]
  [P_BHAL_CAN2_outputs_BHAL_CAN2_outputs_Tag] -> SWC_HALIN_CDD/5
  [P_BHAL_CAN2_outputs_BHAL_CAN2_outputs_Tag] -> SWC_INP/3
  HALR_CAN4_zGW_CANRr1_C50_0_CAN4_SG_zGW_CANRr1_C50_0/1 -> [HALR_CAN4_zGW_CANRr1_C50_0_CAN4_SG_zGW_CANRr1_C50_0_Tag]
  [HALR_CAN4_zGW_CANRr1_C50_0_CAN4_SG_zGW_CANRr1_C50_0_Tag] -> SWC_HALIN/31
  [HALR_CAN4_zGW_CANRr1_C50_0_CAN4_SG_zGW_CANRr1_C50_0_Tag] -> SWC_CGW/24
  HALR_CAN4_ZRR_CE100_1_CAN4_SG_ZRR_CE100_1/1 -> [HALR_CAN4_ZRR_CE100_1_CAN4_SG_ZRR_CE100_1_Tag]
  [HALR_CAN4_ZRR_CE100_1_CAN4_SG_ZRR_CE100_1_Tag] -> SWC_HALIN/30
  [HALR_CAN4_ZRR_CE100_1_CAN4_SG_ZRR_CE100_1_Tag] -> SWC_CGW/23
  HALR_CAN4_ZFR_CE100_0_CAN4_SG_ZFR_CE100_0/1 -> [HALR_CAN4_ZFR_CE100_0_CAN4_SG_ZFR_CE100_0_Tag]
  [HALR_CAN4_ZFR_CE100_0_CAN4_SG_ZFR_CE100_0_Tag] -> SWC_HALIN/28
  [HALR_CAN4_ZFR_CE100_0_CAN4_SG_ZFR_CE100_0_Tag] -> SWC_CGW/21
  HALR_CAN4_ZFR_C100_0_CAN4_SG_ZFR_C100_0/1 -> [HALR_CAN4_ZFR_C100_0_CAN4_SG_ZFR_C100_0_Tag]
  [HALR_CAN4_ZFR_C100_0_CAN4_SG_ZFR_C100_0_Tag] -> SWC_HALIN/27
  [HALR_CAN4_ZFR_C100_0_CAN4_SG_ZFR_C100_0_Tag] -> SWC_CGW/19
  HALR_CAN3_TM_MCUSta2_CAN3_SG_TM_MCUSta2/1 -> [HALR_CAN3_TM_MCUSta2_CAN3_SG_TM_MCUSta2_Tag]
  [HALR_CAN3_TM_MCUSta2_CAN3_SG_TM_MCUSta2_Tag] -> SWC_HALIN/25
  [HALR_CAN3_TM_MCUSta2_CAN3_SG_TM_MCUSta2_Tag] -> SWC_CGW/18
  HALR_CAN3_B2V_ST2_CAN3_SG_B2V_ST2/1 -> [HALR_CAN3_B2V_ST2_CAN3_SG_B2V_ST2_Tag]
  [HALR_CAN3_B2V_ST2_CAN3_SG_B2V_ST2_Tag] -> SWC_HALIN/20
  [HALR_CAN3_B2V_ST2_CAN3_SG_B2V_ST2_Tag] -> SWC_CGW/17
  HALR_CAN3_B2V_ST1_CAN3_SG_B2V_ST1/1 -> [HALR_CAN3_B2V_ST1_CAN3_SG_B2V_ST1_Tag]
  [HALR_CAN3_B2V_ST1_CAN3_SG_B2V_ST1_Tag] -> SWC_HALIN/19
  [HALR_CAN3_B2V_ST1_CAN3_SG_B2V_ST1_Tag] -> SWC_CGW/16
  HALR_CAN3_B2V_BattInfo1_CAN3_SG_B2V_BattInfo1/1 -> [HALR_CAN3_B2V_BattInfo1_CAN3_SG_B2V_BattInfo1_Tag]
  [HALR_CAN3_B2V_BattInfo1_CAN3_SG_B2V_BattInfo1_Tag] -> SWC_HALIN/16
  [HALR_CAN3_B2V_BattInfo1_CAN3_SG_B2V_BattInfo1_Tag] -> SWC_CGW/15
  HALR_CAN3_B2TM_Info_CAN3_SG_B2TM_Info/1 -> [HALR_CAN3_B2TM_Info_CAN3_SG_B2TM_Info_Tag]
  [HALR_CAN3_B2TM_Info_CAN3_SG_B2TM_Info_Tag] -> SWC_HALIN/15
  [HALR_CAN3_B2TM_Info_CAN3_SG_B2TM_Info_Tag] -> SWC_CGW/14
  HALR_CAN1_TC1_CAN1_SG_TC1/1 -> [HALR_CAN1_TC1_CAN1_SG_TC1_Tag]
  [HALR_CAN1_TC1_CAN1_SG_TC1_Tag] -> SWC_HALIN/13
  [HALR_CAN1_TC1_CAN1_SG_TC1_Tag] -> SWC_CGW/9
  HALR_CAN1_HRW_CAN1_SG_HRW/1 -> [HALR_CAN1_HRW_CAN1_SG_HRW_Tag]
  [HALR_CAN1_HRW_CAN1_SG_HRW_Tag] -> SWC_HALIN/12
  [HALR_CAN1_HRW_CAN1_SG_HRW_Tag] -> SWC_CGW/8
  HALR_CAN1_ECAS_DM1_CAN1_SG_ECAS_DM1/1 -> [HALR_CAN1_ECAS_DM1_CAN1_SG_ECAS_DM1_Tag]
  [HALR_CAN1_ECAS_DM1_CAN1_SG_ECAS_DM1_Tag] -> SWC_HALIN/10
  [HALR_CAN1_ECAS_DM1_CAN1_SG_ECAS_DM1_Tag] -> SWC_CGW/7
  HALR_CAN1_EBC1_CAN1_SG_EBC1/1 -> [HALR_CAN1_EBC1_CAN1_SG_EBC1_Tag]
  [HALR_CAN1_EBC1_CAN1_SG_EBC1_Tag] -> SWC_HALIN/7
  [HALR_CAN1_EBC1_CAN1_SG_EBC1_Tag] -> SWC_CGW/6
  HALR_CAN1_ASC1_A_CAN1_SG_ASC1_A/1 -> [HALR_CAN1_ASC1_A_CAN1_SG_ASC1_A_Tag]
  [HALR_CAN1_ASC1_A_CAN1_SG_ASC1_A_Tag] -> SWC_HALIN/6
  [HALR_CAN1_ASC1_A_CAN1_SG_ASC1_A_Tag] -> SWC_CGW/5
  HALR_CAN1_AC_BTMS_C5000_0_CAN1_SG_AC_BTMS_C5000_0/1 -> [HALR_CAN1_AC_BTMS_C5000_0_CAN1_SG_AC_BTMS_C5000_0_Tag]
  [HALR_CAN1_AC_BTMS_C5000_0_CAN1_SG_AC_BTMS_C5000_0_Tag] -> SWC_HALIN/5
  [HALR_CAN1_AC_BTMS_C5000_0_CAN1_SG_AC_BTMS_C5000_0_Tag] -> SWC_CGW/4
  HALR_CAN1_AC_BTMS_C1000_1_CAN1_SG_AC_BTMS_C1000_1/1 -> [HALR_CAN1_AC_BTMS_C1000_1_CAN1_SG_AC_BTMS_C1000_1_Tag]
  [HALR_CAN1_AC_BTMS_C1000_1_CAN1_SG_AC_BTMS_C1000_1_Tag] -> SWC_HALIN/3
  [HALR_CAN1_AC_BTMS_C1000_1_CAN1_SG_AC_BTMS_C1000_1_Tag] -> SWC_CGW/2
  Ground_1/1 -> SWC_HALIN_CDD/4
  SWC_HALOUT/1 -> Terminator_1/1
  SWC_HALOUT/16 -> Terminator_2/1
